simulink library "libbha_kinetic_cc"  (R2013b)
settings: Solver=FixedStepDiscrete  StartTime=0.0  StopTime=Inf  FixedStep=0.004  RelTol=1e-3
PostLoadFcn:
  | , if any(exist('dsrtsu_mdlpostloadfcn', 'file') == [2, 3, 6]), try dsrtsu_mdlpostloadfcn('Execute', bdroot); catch fprintf('Error in PostLoadFcn (dsrtsu_mdlpostloadfcn) for model "%s":\n %s\n', bdroot, lasterr); end, end,
libraries: libbha_parts_bellows x2
(part 4 of 4)

== matlab function libbha_kinetic_cc/lib_ksim_forces_mix_S1/kff_forces_S1 ==
  data: q input size=3; dq input size=3; p input size=3; p_static input size=3; F_ik_Pressure output size=[3,1]; PAR_d_Balg input size=1; PAR_r_Bi input size=1; PAR_b_23 input size=[2,3]; PAR_A_Pressure input size=1; PAR_pAmb input size=1; F_ik_Spring output size=[3,1]; F_ik_Damper output size=[3,1]; F_ik_Bending output size=[3,1]
function [F_ik_Pressure, F_ik_Spring, F_ik_Damper, F_ik_Bending]  = kff_forces(q, dq, p, p_static, PAR_d_Balg, PAR_r_Bi, PAR_b_23, PAR_A_Pressure, PAR_pAmb)
%
% Parameter
%   - [unused]          Schalter zum Definieren der Modi
%   - PAR_A_Pressure    Wirksame Fläche der Druckkraft (sektionsweise)
%   - PAR_D_Balg        Dämpfungsparameter (sektionsweise)
%   - PAR_pAmb          Umgebungsdruck

    %#codegen
    
    %% Druckkraft
    F_ik_Pressure = (p - PAR_pAmb) .* PAR_A_Pressure(1);
    
    %% Dämperkraft
    F_ik_Damper   = dq .* PAR_d_Balg(1);
    
    %% Federkraft 
    F_ik_Spring = PAR_A_Pressure(1).* p_static;
    
    %% Biegekraft 
    % neue Biegekraftberechnung
    k                 = calc_k_i(q(1), q(2), q(3), PAR_r_Bi); % phi1; kappa1; ell1   
                      
    F_ik_Bending = fcn_getpbend(k(1,:), k(2,:), k(3,:), PAR_b_23) .* PAR_A_Pressure; 
    
    
    
end


% D:\Dokumente\Projekte\Festo-BHA\23 Messergebnisse\Federkennlinie (Identifizierung) (2015-06) ISYS
function p_bend = fcn_getpbend(phi, kappa, ell, PAR_kl_gain) 
    % phi   = [1 x n]
    % kappa = [1 x n]
    % ell   = [1 x n]
    % PAR_kl_gain = [2 x 3*n] mit [2 x 3] = [M1:1 M2:1 M3:1; M1:2 M2:2 M3:2]'
    %               (erste Zeile: Einzelbälge, zweite Zeile Doppelbälge)
    
    % vektorielle Eingänge gelten für 3 Sektionen
    % Phi muss als Spaltenvektor (eine Zeile) vorliegen
    
    %% Bestimmung der Phi-Projektion des aufgeteilten Phi-Kreises
    [iStart,iEnd,tcos] = fcn_split_phi(phi); % für jedes Phi Start- und End-Indices mit Gewichtungsverhältnis (tcos) berechnen
    % Start- und Endindex/Messzuweisung pro Sektion/Phi: 
    % abs(.) -> Messnummer (Einzelbalg i gegen restlichen Doppelbalg)
    % sign(.) -> Vorzeichen (+kappa/-kappa)
    % Kurve 1 oder 2 aus 2-(Balgnummer==abs(Messzuweisung);
    
    %% Für jede Sektion entsprechende Zeilen aus PAR_kl_gain auswählen
    %       111   121   131   211   221   231   311   321   331  <-- PAR_kl_gain
    %       112   122   132   212   222   232   312   322   332
    %       ---------------   ---------------   ---------------  <-- iStart-Index wähl von jedem Block die i-te Spalte aus
        
    valStart = PAR_kl_gain(:,abs(iStart)) .* ([1;1]*(sign(iStart).*kappa.*ell));
    valEnd   = PAR_kl_gain(:,abs(iEnd)  ) .* ([1;1]*(sign(iEnd  ).*kappa.*ell)); 
    
    % Zwei Ergebnisse der beiden Parameterkurven auf drei Bälge übertragen
    % Matrix: Zeilen entsprechen den Bälgen, Spalten den Sektionen
    %   Indizierung: erster Teil Balgzuweisungen (aus 1 oder 2) pro Sektion,
    %                zweiter Teil: Skalierung auf Gesamtindices
        
    pStart   = valStart( 2-([1;2;3]-abs(iStart)==0) );
    pEnd     = valEnd(   2-([1;2;3]-abs(iEnd  )==0) );
    
    delta = (pEnd - pStart)/2;
    mw    = (pEnd + pStart)/2;
    
    % Cosinus-Interpolation zwischen Start und Ende (mittels Mittelwert und Delta)
    p_bend   = -delta.*cos([1;1;1]*tcos) + mw;
    
end

function [iStart,iEnd,tcos] = fcn_split_phi(phi)
    %% Rückgabe:
    %       iStart: [1xlenphi]  (früher [3xlenphi])
    %       iEnd:   [1xlenphi]  (früher [3xlenphi])
    %       tcos:   [1xlenphi] <-- ggf auch transponiert, wenn phi nicht [1xX]

    %% Aufteilung des Phi-Kreises in 6 Bereiche         Balg 1      Balg 2      Balg 3
    % 0   .. 1/3 pi  --  Krümmung zu (1)                +M1:1		+M1:2		+M1:2
    % 1/3 .. 2/3 pi  --  Krümmung zu (1-2)              -M3:2       -M3:2       -M3:1
    % 2/3 .. 1   pi  --  Krümmung zu (2)                +M2:2       +M2:1       +M2:2
    % 1   .. 4/3 pi  --  Krümmung zu (2-3)              -M1:1       -M1:2       -M1:2
    % 4/3 .. 5/3 pi  --  Krümmung zu (3)                +M3:2       +M3:2       +M3:1
    % 5/3 .. 2   pi  --  Krümmung zu (3-1)              -M2:2       -M2:1       -M2:2

    % Indexzuweisungen: jew. Messungen für verschiedene Phasen
    Messzuweisung = [ +1, -3, +2, -1, +3, -2]; % ob Kurve 1 oder 2 ergibt sich aus 2-(Balgnummer==abs(Messzuweisung);
    
    %% Cosinus-Interpolation zwischen allen Start- und Endvektoren
    % liefert Startindex (1-6) und Endindex
    tcos = mod((phi*3),pi); % arg(cos) zwischen 0 und pi
    %tcos = mod((phi/pi),1/3)*3*pi; %% gleiches Ergebnis
    
    %% Phi-abhängige Auswahl der 6 Bereiche für alle drei Bälge
    % sel_idx   = mod([1;1;1]*round((3*phi-tcos)/pi)+([1;5;3]-1)*ones(1,size(phi,2)),6)+1;   % Formel: Zeileneintrag für jeden Balg, phi muss als Zeilenvektor (horizontal) vorliegen (ein Eintrag pro Sektion)
    sel_idx   = mod(round((3*phi-tcos)/pi),6)+1;                                             % Formel: nur ein Zeileneintrag,        phi kann als Zeilenvektor (horizontal) vorliegen (ein Eintrag pro Sektion)
    
    iStart = Messzuweisung(sel_idx);
    iEnd   = Messzuweisung(mod(sel_idx,6)+1);
    
end


%%  Konfigurationszustand k = [phi, kappa, ell]^T 
% aus: libbha_kinetic_cc\lib_kinm

%  Konfigurationszustand einer Sektion 
function [k_i] = calc_k_i(q1,q2,q3, d)
    % Input:
    %   - qi = [ell_i1, ell_i2, ell_i3]^T       Aktorzustand
    %   - d                                     Radialer Abstand der Aktorsymmetrielinie  
    %
    % Output:
    %   - ki   [3 x 1]                          Konfigurationszustand 

    % Vermeidung Singularität
    qist_eps  = 1e-15;
    qist      = q1.^2 + q2.^2 + q3.^2 - q1.*q2 - q1.*q3 - q2.*q3;
    while (qist<qist_eps)
        q1      = q1 - 5e-8;
        qist  = q1.^2 + q2.^2 + q3.^2 - q1.*q2 - q1.*q3 - q2.*q3;
    end

    % Substitutionen
    q_sum   = q1 + q2 + q3;
    
    % Konfigurationszustand
    mphi    = atan2(sqrt(0.3e1) * (q3-q2) , (q2+q3 - 2*q1));
    mkappa  = 2.0 * sqrt(qist) / (d*q_sum);
    mell    = (q1 + q2 + q3)/3.0;
    
    k_i = [mphi;
           mkappa;
           mell];
end
